simulink model "PIDuRelayy"  (R2021b)
settings: Solver=FixedStepAuto  StartTime=0.0  StopTime=5000  FixedStep=0.2  RelTol=1e-3
undefined symbols (not defined in the file or in its folder): setsin
settings Model: Creator=ismt  LastModifiedBy=ismt

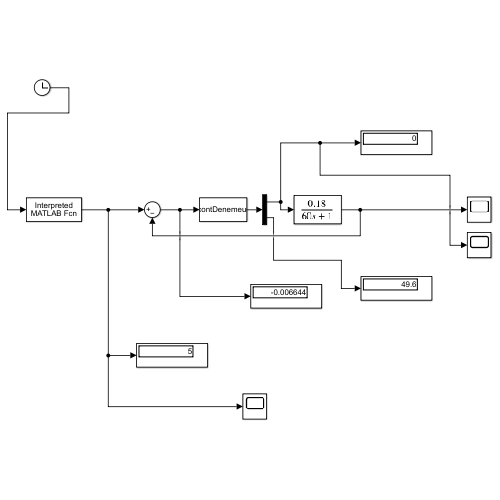
[thumbnail: Simulink's stored preview of the top-level diagram]
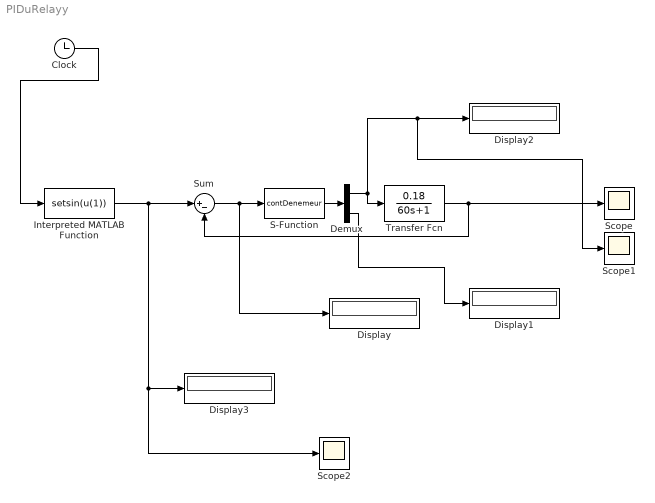
== system PIDuRelayy ==
  Clock : Clock
  Demux : Demux  Outputs=2
  Display{,1..3} (4 alike) : Display
  Interpreted MATLAB Function : MATLABFcn  MATLABFcn=setsin(u(1))
  S-Function : S-Function  FunctionName=contDenemeur  SFunctionDeploymentMode=off  EnableBusSupport=off
  Scope : Scope
  Scope1 : Scope
  Scope2 : Scope
  Sum : Sum  Inputs=|+-
  Transfer Fcn : TransferFcn  Numerator=[0.18]  Denominator=[60 1]
  wires:
  Sum/1 -> Display/1, S-Function/1
  Interpreted MATLAB Function/1 -> Scope2/1, Display3/1, Sum/1
  Transfer Fcn/1 -> Scope/1, Sum/2
  S-Function/1 -> Demux/1
  Demux/1 -> Scope1/1, Display2/1, Transfer Fcn/1
  Demux/2 -> Display1/1
  Clock/1 -> Interpreted MATLAB Function/1
